simulink model "semi6_2_indirect"  (R2023a)
settings: Solver=VariableStepAuto  StartTime=0.0  StopTime=0.2  MaxStep=1e-5  RelTol=1e-3
libraries: spsIGBTDiodeLib x4, spsFourierLib x2, spsRMSLib x2, spsVoltageMeasurementLib x2, spsACVoltageSourceLib x1, spsDCVoltageSourceLib x1, spsCurrentMeasurementLib x1, spsSeriesRLCBranchLib x1, spsTriangleGeneratorLib x1, spspowerguiLib x1
settings Model: Creator=小刘  LastModifiedBy=11094
settings DataIOCC: ReturnWorkspaceOutputs=off
settings OptimizationCC: ReuseModelBlockBuffer=off
settings DebuggingCC: UnconnectedInputMsg=warning  UnconnectedOutputMsg=warning  UnconnectedLineMsg=warning
settings ModelReferenceCC: EnableRefExpFcnMdlSchedulingChecks=on
settings RTWCC: DLArmComputeVersion=19.05

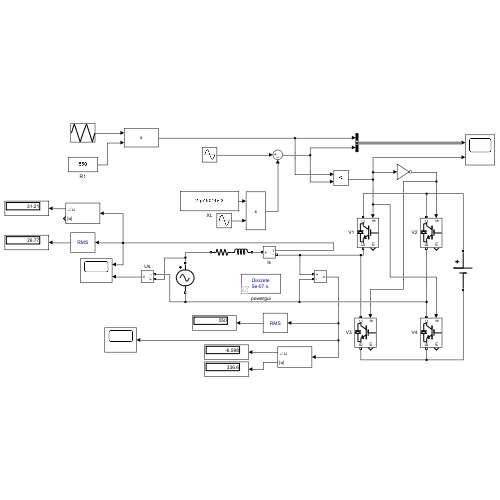
[thumbnail: Simulink's stored preview of the top-level diagram]
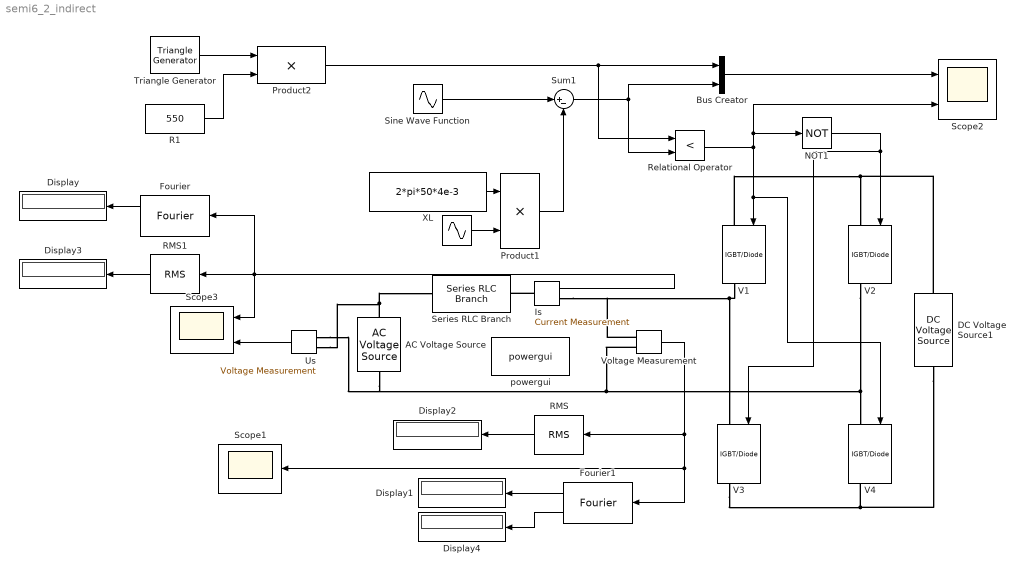
== system semi6_2_indirect ==
  " " : Sin  Amplitude=25*sqrt(2)  Frequency=2*pi*50  Phase=30*pi/180+pi/2  SampleTime=0
  AC Voltage Source : spsACVoltageSourceLib/AC Voltage Source  Amplitude=220*sqrt(2)  Phase=0  Frequency=50  SampleTime=0  Measurements=None  BusType=swing  Pref=10e3  Qref=0  Qmin=-inf  Qmax=+inf
  Bus Creator : BusCreator  Inputs=2
  DC Voltage Source1 : spsDCVoltageSourceLib/DC Voltage Source  Amplitude=550  Measurements=None
  Display{,1..4} (5 alike) : Display
  Fourier : spsFourierLib/Fourier  Freq=50  n=1  InInit=[0, 0]  Ts=0
  Fourier1 : spsFourierLib/Fourier  Freq=50  n=1  InInit=[0, 0]  Ts=0
  Is : spsCurrentMeasurementLib/Current Measurement  PhasorSimulation=off  OutputType=Complex  PSBequivalent=0
  NOT1 : Logic  Operator=NOT  IconShape=distinctive  AllPortsSameDT=off  OutDataTypeStr=boolean
  Product1 : Product
  Product2 : Product
  R1 : Constant  Value=550
  RMS : spsRMSLib/RMS  TrueRMS=on  Freq=60  RMSInit=120  Ts=0
  RMS1 : spsRMSLib/RMS  TrueRMS=on  Freq=50  RMSInit=120  Ts=0
  Relational Operator : RelationalOperator  Operator=<  OutDataTypeStr=boolean  RndMeth=Simplest  InputSameDT=off
  Scope1 : Scope
  Scope2 : Scope  NumInputPorts=2
  Scope3 : Scope  NumInputPorts=2
  Series RLC Branch : spsSeriesRLCBranchLib/Series RLC Branch  LConnTagsString=__new0  RConnTagsString=__new0  BranchType=RL  Resistance=0  Inductance=4e-3  SetiL0=off  InitialCurrent=0  Capacitance=1e-6  Setx0=off  InitialVoltage=0  Measurements=None
  Sine Wave Function : Sin  Amplitude=220*sqrt(2)  Frequency=2*pi*50  SampleTime=0
  Sum1 : Sum  Inputs=|+-
  Triangle Generator : spsTriangleGeneratorLib/Triangle Generator  Freq=20e3  Phase=90  Ts=0
  Us : spsVoltageMeasurementLib/Voltage Measurement  PhasorSimulation=off  OutputType=Complex  PSBequivalent=0
  V{1..4} (4 alike) : spsIGBTDiodeLib/IGBT//Diode  Ron=1e-3  Rs=1e5  Cs=inf  Measurements=on
  Voltage Measurement : spsVoltageMeasurementLib/Voltage Measurement  PhasorSimulation=off  OutputType=Complex  PSBequivalent=0
  XL : Constant  Value=2*pi*50*4e-3
  powergui : spspowerguiLib/powergui  Priority=1  SimulationMode=Discrete  SampleTime=50e-8  frequency=60  Iterations=50  frequencyindice=50  Pbase=100e6  ErrMax=1e-4  UnitsV=kV  UnitsW=MW  buscounter=0  FunctionMessages=off  echomessages=off  EnableUseOfTLC=off  CurrentSourceSwitches=off  DisableSnubberDevices=off  DisableRonSwitches=off  DisableVfSwitches=off  DisplayEquations=off  AutomaticDiscreteSolvers=off  SolverType=Tustin/Backward Euler (TBE)  Interpol=off  ExternalGateDelay=off  methode=off  Ts=100  x0status=blocks  SPID=on  SwTol=0  HookPort=off  NonlinearTolerance=1e-4  nMaxIteration=100  ContinueOnMaxIteration=off  RestoreLinks=warning  ResistiveCurrentMeasurement=off  Frange=[0:2:500]  Ylog=off  Xlog=on  ShowGrid=off  save=off  variable=ZData  structure=0  ZoomFFT=off  StartTime=0.0  cycles=1  DisplayStyle=1  fundamental=60  FreqAxis=off  MaxFrequency=1000  frequencyindicesteady=1  RmsSteady=1  display=off
  wires:
  " "/1 -> Product1/2
  Sine Wave Function/1 -> Sum1/1
  Product1/1 -> Sum1/2
  Sum1/1 -> Bus Creator/2, Relational Operator/2
  Triangle Generator/1 -> Product2/1
  R1/1 -> Product2/2
  Product2/1 -> Relational Operator/1, Bus Creator/1
  Relational Operator/1 -> Scope2/2, NOT1/1, V4/1, V1/1
  NOT1/1 -> V3/1, V2/1
  Fourier/2 -> Display/1
  Is/1 -> Fourier/1, Scope3/1, RMS1/1
  XL/1 -> Product1/1
  Voltage Measurement/1 -> Scope1/1, Fourier1/1, RMS/1
  RMS/1 -> Display2/1
  RMS1/1 -> Display3/1
  Bus Creator/1 -> Scope2/1
  Us/1 -> Scope3/2
  Fourier1/2 -> Display1/1
  Fourier1/1 -> Display4/1
  connections:
  V3/RConn1 -- DC Voltage Source1/LConn1 -- V4/RConn1
  V2/RConn1 -- Us/LConn2 -- AC Voltage Source/LConn1 -- Voltage Measurement/LConn2 -- V4/LConn1
  V1/RConn1 -- Is/RConn1 -- Voltage Measurement/LConn1 -- V3/LConn1
  V1/LConn1 -- DC Voltage Source1/RConn1 -- V2/LConn1
  AC Voltage Source/RConn1 -- Series RLC Branch/LConn1 -- Us/LConn1
  Is/LConn1 -- Series RLC Branch/RConn1
